simulink model "SF011A_EotLrng"  (R2013b)
settings: Solver=FixedStepDiscrete  SolverMode=SingleTasking  StartTime=0.0  StopTime=1  FixedStep=0.002  RelTol=1e-3
values from neighbouring files (symbols this model uses):
  ARCHGLBPRM_FLOATZEROTHD_ULS_F32 = DataDict.Constant    [SF011A_EotLrng_DataDict.m]
  CNVTOMILLISEC_MILLISECPERCNT_F32 = DataDict.Constant    [SF011A_EotLrng_DataDict.m]
  CORRLNFLT_CNT_U08 = DataDict.Constant    [SF011A_EotLrng_DataDict.m]
  DEBSTEP_CNT_U16 = DataDict.Constant    [SF011A_EotLrng_DataDict.m]
  EOTLIMDETD_CNT_LOGL = DataDict.Constant    [SF011A_EotLrng_DataDict.m]
  EOTLIMNOTDETD_CNT_LOGL = DataDict.Constant    [SF011A_EotLrng_DataDict.m]
  EotLrngAuthyStrtLrn = DataDict.Calibration    [SF011A_EotLrng_DataDict.m]
  EotLrngEotLrnTmr = DataDict.Calibration    [SF011A_EotLrng_DataDict.m]
  EotLrngHwAgOverTrvlCnt = DataDict.Calibration    [SF011A_EotLrng_DataDict.m]
  EotLrngHwAgOverTrvlEntr = DataDict.Calibration    [SF011A_EotLrng_DataDict.m]
  EotLrngHwAgOverTrvlExit = DataDict.Calibration    [SF011A_EotLrng_DataDict.m]
  EotLrngHwTqEotLrn = DataDict.Calibration    [SF011A_EotLrng_DataDict.m]
  EotLrngMotVelEotLrn = DataDict.Calibration    [SF011A_EotLrng_DataDict.m]
  EotLrngRackTrvlMax = DataDict.Calibration    [SF011A_EotLrng_DataDict.m]
  EotLrngRackTrvlMin = DataDict.Calibration    [SF011A_EotLrng_DataDict.m]
  EotLrngRstAuthyMin = DataDict.Calibration    [SF011A_EotLrng_DataDict.m]
  EotProtnRackTrvlLimrEna = DataDict.ImprtdCal    [SF011A_EotLrng_DataDict.m]
  HwAgOverTrvl = DataDict.NTC    [SF011A_EotLrng_DataDict.m]
  HWAGOVERTRVLMAXCNT_CNT_U08 = DataDict.Constant    [SF011A_EotLrng_DataDict.m]
  NODEBSTEP_CNT_U16 = DataDict.Constant    [SF011A_EotLrng_DataDict.m]
  OUTOFRNGFLT_CNT_U08 = DataDict.Constant    [SF011A_EotLrng_DataDict.m]
  RackEotStorgFlt = DataDict.NTC    [SF011A_EotLrng_DataDict.m]
  SIGAVLFLT_CNT_U08 = DataDict.Constant    [SF011A_EotLrng_DataDict.m]
undefined symbols (not defined in the file or in its folder): NtcSts1, NvmGetErrSts1, SigQlfr1
libraries: simulink x19, NxtrNvM x12, NxtrAbslt x5, NxtrLim x4, NxtrMax x3, NxtrMin x3
(part 2 of 7)

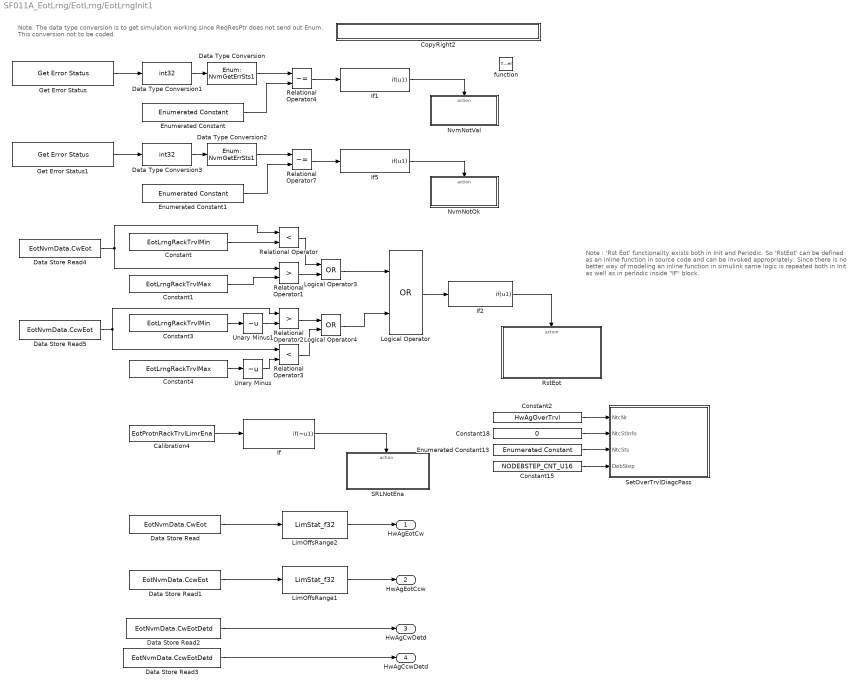
== system SF011A_EotLrng/EotLrng/EotLrngInit1 ==
  note: Note: The data type conversion is to get simulation working since ReqResPtr does not send out Enum. This
      | conversion not to be coded.
  note: Note : 'Rst Eot' functionality exists both in Init and Periodic.
      | So 'RstEot' can be defined as an inline function in source code and can be invoked
      | appropriately. Since there is no better way of modeling an inline function in simulink
      | same logic is repeated both in Init as well as in periodic inside "IF" block.
  function : TriggerPort  TriggerType=function-call
  Calibration4 : Constant  RequirementInfo="{'linktype_rmi_doors' '0000ba59 (/E-STEER Core/SubSystem Specifications/Application Functions/SF011A Learned EOT Limits)' '#SF011A_125' 'true' 'REQ:  SF011A_125' '' } %GIDa_8cd91484_508f_4a19_9e50_6e4bd6d6bfd9"  Value=EotProtnRackTrvlLimrEna
  Constant : Constant  RequirementInfo="{'linktype_rmi_doors' '0000ba59 (/E-STEER Core/SubSystem Specifications/Application Functions/SF011A Learned EOT Limits)' '#SF011A_70' 'true' 'REQ:  SF011A_70' '' ; 'linktype_rmi_doors' '0000ba59 (/E-STEER Core/SubSystem Specifications/Application Functions/SF011A Learned EOT Limits)' '#SF011A_48' 'true' 'REQ:  SF011A_48' '' } %GIDa_a6aa3c9d_e3af_4644_902f_5becbbdfb912"  Value=EotLrngRackTrvlMin
  Constant1 : Constant  RequirementInfo="{'linktype_rmi_doors' '0000ba59 (/E-STEER Core/SubSystem Specifications/Application Functions/SF011A Learned EOT Limits)' '#SF011A_70' 'true' 'REQ:  SF011A_70' '' ; 'linktype_rmi_doors' '0000ba59 (/E-STEER Core/SubSystem Specifications/Application Functions/SF011A Learned EOT Limits)' '#SF011A_49' 'true' 'REQ:  SF011A_49' '' } %GIDa_a0828fd1_c5cb_4d17_a3e1_4c408a8731ec"  Value=EotLrngRackTrvlMax
  Constant15 : Constant  RequirementInfo={} %GIDa_e57038bb_d9c8_49ea_a4b9_f6e761d5e128  Value=NODEBSTEP_CNT_U16
  Constant18 : Constant  RequirementInfo={} %GIDa_4611f9eb_ed4b_4f11_915a_23b80d8496d3  Value=0
  Constant2 : Constant  RequirementInfo={} %GIDa_c7caa921_f92d_4602_b505_ea668ad6087d  Value=HwAgOverTrvl
  Constant3 : Constant  RequirementInfo="{'linktype_rmi_doors' '0000ba59 (/E-STEER Core/SubSystem Specifications/Application Functions/SF011A Learned EOT Limits)' '#SF011A_71' 'true' 'REQ:  SF011A_71' '' ; 'linktype_rmi_doors' '0000ba59 (/E-STEER Core/SubSystem Specifications/Application Functions/SF011A Learned EOT Limits)' '#SF011A_48' 'true' 'REQ:  SF011A_48' '' } %GIDa_5f1678bd_b67c_4df4_9938_38fbe269600f"  Value=EotLrngRackTrvlMin
  Constant4 : Constant  RequirementInfo="{'linktype_rmi_doors' '0000ba59 (/E-STEER Core/SubSystem Specifications/Application Functions/SF011A Learned EOT Limits)' '#SF011A_71' 'true' 'REQ:  SF011A_71' '' ; 'linktype_rmi_doors' '0000ba59 (/E-STEER Core/SubSystem Specifications/Application Functions/SF011A Learned EOT Limits)' '#SF011A_49' 'true' 'REQ:  SF011A_49' '' } %GIDa_30774794_edea_413e_bdbc_5a0164b2a6d6"  Value=EotLrngRackTrvlMax
  CopyRight2 : Subsystem  Description=|  mask(Copyright Information){none=on}
      | Copyright info block.                                               
      |                                                                     
      | Place copyright information at the top of every subsystem in design.
      mask prompts: none "No parameters"
      mask help: Place copyright information at the top of every subsystem in design.
      mask Display:
      | NxtrConf = 'Nexteer Confidential';
      | 
      | sys = bdroot; %handle for the current model ("system")
      | first = get_param(sys,'Created');
      | if(isempty(first))
      |     first = datestr(now,'yyyy');
      | else
      |     first = first(end-3:end);  %year is last four digits
      | end
      | 
      | last = get_param(sys,'LastModifiedDate');
      | if isempty(last)
      |     last = datestr(now,'yyyy');
      | else
      |     last = last(end-3:end);
      | end
      | 
      | if strcmp(first,last)
      |     fprintf('%s -- Copyright %s Nexteer',NxtrConf,first)
      | else
      |     fprintf('%s -- %s%s- %s Nexteer',NxtrConf,char(169),first,last)
      | end
  Data Store Read : DataStoreRead  RequirementInfo="{'linktype_rmi_doors' '0000ba59 (/E-STEER Core/SubSystem Specifications/Application Functions/SF011A Learned EOT Limits)' '#SF011A_60' 'true' 'REQ:  SF011A_60' '' ; 'linktype_rmi_doors' '0000ba59 (/E-STEER Core/SubSystem Specifications/Application Functions/SF011A Learned EOT Limits)' '#SF011A_59' 'true' 'REQ:  SF011A_59' '' ; 'linktype_rmi_doors' '0000ba59 (/E-STEER Core/SubSystem Specifications/Application Functions/SF011A Learned EOT Limits)' '#SF011A_72' 'true' 'REQ:  SF011A_72' '' } %GIDa_1cce3593_98c7_4927_96ef_8fd09f8c13ce"  DataStoreName=EotNvmData  DataStoreElements=EotNvmData.CwEot
  Data Store Read1 : DataStoreRead  RequirementInfo="{'linktype_rmi_doors' '0000ba59 (/E-STEER Core/SubSystem Specifications/Application Functions/SF011A Learned EOT Limits)' '#SF011A_61' 'true' 'REQ:  SF011A_61' '' ; 'linktype_rmi_doors' '0000ba59 (/E-STEER Core/SubSystem Specifications/Application Functions/SF011A Learned EOT Limits)' '#SF011A_59' 'true' 'REQ:  SF011A_59' '' ; 'linktype_rmi_doors' '0000ba59 (/E-STEER Core/SubSystem Specifications/Application Functions/SF011A Learned EOT Limits)' '#SF011A_73' 'true' 'REQ:  SF011A_73' '' } %GIDa_59ef2486_936c_413c_9940_c67c54ecfdbd"  DataStoreName=EotNvmData  DataStoreElements=EotNvmData.CcwEot
  Data Store Read2 : DataStoreRead  RequirementInfo="{'linktype_rmi_doors' '0000ba59 (/E-STEER Core/SubSystem Specifications/Application Functions/SF011A Learned EOT Limits)' '#SF011A_62' 'true' 'REQ:  SF011A_62' '' ; 'linktype_rmi_doors' '0000ba59 (/E-STEER Core/SubSystem Specifications/Application Functions/SF011A Learned EOT Limits)' '#SF011A_59' 'true' 'REQ:  SF011A_59' '' ; 'linktype_rmi_doors' '0000ba59 (/E-STEER Core/SubSystem Specifications/Application Functions/SF011A Learned EOT Limits)' '#SF011A_74' 'true' 'REQ:  SF011A_74' '' } %GIDa_37d3043a_15c7_4be1_94c6_67c59661e3c0"  DataStoreName=EotNvmData  DataStoreElements=EotNvmData.CwEotDetd
  Data Store Read3 : DataStoreRead  RequirementInfo="{'linktype_rmi_doors' '0000ba59 (/E-STEER Core/SubSystem Specifications/Application Functions/SF011A Learned EOT Limits)' '#SF011A_63' 'true' 'REQ:  SF011A_63' '' ; 'linktype_rmi_doors' '0000ba59 (/E-STEER Core/SubSystem Specifications/Application Functions/SF011A Learned EOT Limits)' '#SF011A_59' 'true' 'REQ:  SF011A_59' '' ; 'linktype_rmi_doors' '0000ba59 (/E-STEER Core/SubSystem Specifications/Application Functions/SF011A Learned EOT Limits)' '#SF011A_75' 'true' 'REQ:  SF011A_75' '' } %GIDa_cb0e143f_3fff_4146_ad36_117712b20001"  DataStoreName=EotNvmData  DataStoreElements=EotNvmData.CcwEotDetd
  Data Store Read4 : DataStoreRead  RequirementInfo="{'linktype_rmi_doors' '0000ba59 (/E-STEER Core/SubSystem Specifications/Application Functions/SF011A Learned EOT Limits)' '#SF011A_70' 'true' 'REQ:  SF011A_70' '' } %GIDa_1f2eef30_41ac_4ca5_aa34_dae99e9f45ec"  DataStoreName=EotNvmData  DataStoreElements=EotNvmData.CwEot
  Data Store Read5 : DataStoreRead  RequirementInfo="{'linktype_rmi_doors' '0000ba59 (/E-STEER Core/SubSystem Specifications/Application Functions/SF011A Learned EOT Limits)' '#SF011A_71' 'true' 'REQ:  SF011A_71' '' } %GIDa_ec91acdb_3367_426b_b3a6_fca3d2bebdb1"  DataStoreName=EotNvmData  DataStoreElements=EotNvmData.CcwEot
  Data Type Conversion : DataTypeConversion  RequirementInfo="{'linktype_rmi_doors' '0000ba59 (/E-STEER Core/SubSystem Specifications/Application Functions/SF011A Learned EOT Limits)' '#SF011A_124' 'true' 'REQ:  SF011A_124' '' } %GIDa_40e4bb70_1115_4c40_912d_1afd6378f698"  OutDataTypeStr=Enum: NvmGetErrSts1
  Data Type Conversion1 : DataTypeConversion  RequirementInfo="{'linktype_rmi_doors' '0000ba59 (/E-STEER Core/SubSystem Specifications/Application Functions/SF011A Learned EOT Limits)' '#SF011A_124' 'true' 'REQ:  SF011A_124' '' } %GIDa_af9c1c5f_4576_4c81_a62f_597d688de759"  OutDataTypeStr=int32
  Data Type Conversion2 : DataTypeConversion  RequirementInfo="{'linktype_rmi_doors' '0000ba59 (/E-STEER Core/SubSystem Specifications/Application Functions/SF011A Learned EOT Limits)' '#SF011A_124' 'true' 'REQ:  SF011A_124' '' } %GIDa_9c8c0f48_10fc_41fa_ac24_1a39867ed0ea"  OutDataTypeStr=Enum: NvmGetErrSts1
  Data Type Conversion3 : DataTypeConversion  RequirementInfo="{'linktype_rmi_doors' '0000ba59 (/E-STEER Core/SubSystem Specifications/Application Functions/SF011A Learned EOT Limits)' '#SF011A_124' 'true' 'REQ:  SF011A_124' '' } %GIDa_ea8dac4b_68c0_40a2_8dd8_c1010ce976e9"  OutDataTypeStr=int32
  Enumerated Constant13 : simulink/Sources/Enumerated Constant  RequirementInfo={} %GIDa_38909906_b1fb_4b03_8f37_3dee4a706b69  OutDataTypeStr=Enum: NtcSts1  Value=NtcSts1.NTCSTS_PASSD  SampleTime=inf
  Enumerated Constant : simulink/Sources/Enumerated Constant  RequirementInfo="{'linktype_rmi_doors' '0000ba59 (/E-STEER Core/SubSystem Specifications/Application Functions/SF011A Learned EOT Limits)' '#SF011A_124' 'true' 'REQ:  SF011A_124' '' } %GIDa_af7030e8_a7a1_47be_8aa5_0a8feabfae11"  OutDataTypeStr=Enum: NvmGetErrSts1  Value=NvmGetErrSts1.REQUEST_OK  SampleTime=inf
  Enumerated Constant1 : simulink/Sources/Enumerated Constant  RequirementInfo="{'linktype_rmi_doors' '0000ba59 (/E-STEER Core/SubSystem Specifications/Application Functions/SF011A Learned EOT Limits)' '#SF011A_124' 'true' 'REQ:  SF011A_124' '' } %GIDa_38a139b3_f8e9_4563_8a22_5346e1b58213"  OutDataTypeStr=Enum: NvmGetErrSts1  Value=NvmGetErrSts1.REQUEST_OK  SampleTime=inf
  Get Error Status : NxtrNvM/Get Error Status  RequirementInfo="{'linktype_rmi_doors' '0000ba59 (/E-STEER Core/SubSystem Specifications/Application Functions/SF011A Learned EOT Limits)' '#SF011A_124' 'true' 'REQ:  SF011A_124' '' } %GIDa_295c35b2_dd27_46e5_9350_5c6db25722f0"  FuncName=Get Error Status  NvMBlockName=EotNvmData  VoidFuncRtn=on  ReqResPtr_DSN=NvMReqResPtr  Return_DSN=NvMGES_ReqResPtr
      settings: AttributesFormatString=%<FuncName>
  Get Error Status1 : NxtrNvM/Get Error Status  RequirementInfo="{'linktype_rmi_doors' '0000ba59 (/E-STEER Core/SubSystem Specifications/Application Functions/SF011A Learned EOT Limits)' '#SF011A_124' 'true' 'REQ:  SF011A_124' '' } %GIDa_5993ad55_5530_455e_9e47_61c827e0bbdf"  FuncName=Get Error Status  NvMBlockName=MaxHwAgCwAndCcw  VoidFuncRtn=on  ReqResPtr_DSN=NvMReqResPtr1  Return_DSN=NvMGES_ReqResPtr1
      settings: AttributesFormatString=%<FuncName>
  If : If  RequirementInfo="{'linktype_rmi_doors' '0000ba59 (/E-STEER Core/SubSystem Specifications/Application Functions/SF011A Learned EOT Limits)' '#SF011A_125' 'true' 'REQ:  SF011A_125' '' } %GIDa_3d6ad9bb_5e78_4a41_a61b_bd13d670cab6"  Priority=2  IfExpression=~u1  ShowElse=off
  If1 : If  RequirementInfo="{'linktype_rmi_doors' '0000ba59 (/E-STEER Core/SubSystem Specifications/Application Functions/SF011A Learned EOT Limits)' '#SF011A_124' 'true' 'REQ:  SF011A_124' '' } %GIDa_91d6c890_e003_4682_8730_094d0138a595"  Priority=0  IfExpression=u1  ShowElse=off
  If2 : If  RequirementInfo="{'linktype_rmi_doors' '0000ba59 (/E-STEER Core/SubSystem Specifications/Application Functions/SF011A Learned EOT Limits)' '#SF011A_70' 'true' 'REQ:  SF011A_70' '' ; 'linktype_rmi_doors' '0000ba59 (/E-STEER Core/SubSystem Specifications/Application Functions/SF011A Learned EOT Limits)' '#SF011A_71' 'true' 'REQ:  SF011A_71' '' } %GIDa_a534ff47_bac3_4be0_88f9_462c603ec428"  Priority=1  IfExpression=u1  ShowElse=off
  If5 : If  RequirementInfo="{'linktype_rmi_doors' '0000ba59 (/E-STEER Core/SubSystem Specifications/Application Functions/SF011A Learned EOT Limits)' '#SF011A_124' 'true' 'REQ:  SF011A_124' '' } %GIDa_8f477629_7324_4566_aadd_9e30a62de6d3"  Priority=0  IfExpression=u1  ShowElse=off
  LimOffsRange1 : NxtrLim/LimStat_f32  RequirementInfo="{'linktype_rmi_doors' '0000ba59 (/E-STEER Core/SubSystem Specifications/Application Functions/SF011A Learned EOT Limits)' '#SF011A_39' 'true' 'REQ:  SF011A_39' '' } %GIDa_51d5d642_7edf_4836_a1f4_3c017c910443"  LoLim=HWAGEOTCCWLOWLIM_HWDEG_F32  HiLim=HWAGEOTCCWHILIM_HWDEG_F32
      settings: AttributesFormatString=|
      | Low Limit: %<LoLim>
      | High Limit:%<HiLim>
  LimOffsRange2 : NxtrLim/LimStat_f32  RequirementInfo="{'linktype_rmi_doors' '0000ba59 (/E-STEER Core/SubSystem Specifications/Application Functions/SF011A Learned EOT Limits)' '#SF011A_11' 'true' 'REQ:  SF011A_11' '' } %GIDa_4df0df7c_5c40_4811_b091_ccf12396757f"  LoLim=HWAGEOTCWLOWLIM_HWDEG_F32  HiLim=HWAGEOTCWHILIM_HWDEG_F32
      settings: AttributesFormatString=|
      | Low Limit: %<LoLim>
      | High Limit:%<HiLim>
  Logical Operator : Logic  RequirementInfo="{'linktype_rmi_doors' '0000ba59 (/E-STEER Core/SubSystem Specifications/Application Functions/SF011A Learned EOT Limits)' '#SF011A_70' 'true' 'REQ:  SF011A_70' '' ; 'linktype_rmi_doors' '0000ba59 (/E-STEER Core/SubSystem Specifications/Application Functions/SF011A Learned EOT Limits)' '#SF011A_71' 'true' 'REQ:  SF011A_71' '' } %GIDa_ebb98ba6_f107_46ce_9d07_fa346759ea33"  Operator=OR  AllPortsSameDT=off  OutDataTypeStr=boolean
  Logical Operator3 : Logic  RequirementInfo="{'linktype_rmi_doors' '0000ba59 (/E-STEER Core/SubSystem Specifications/Application Functions/SF011A Learned EOT Limits)' '#SF011A_70' 'true' 'REQ:  SF011A_70' '' } %GIDa_aaf30ec3_ce61_43e6_b06a_936d4bd8ccf6"  Operator=OR  AllPortsSameDT=off  OutDataTypeStr=boolean
  Logical Operator4 : Logic  RequirementInfo="{'linktype_rmi_doors' '0000ba59 (/E-STEER Core/SubSystem Specifications/Application Functions/SF011A Learned EOT Limits)' '#SF011A_71' 'true' 'REQ:  SF011A_71' '' } %GIDa_33792c4b_275f_4e69_ac68_2ae50f8c8a65"  Operator=OR  AllPortsSameDT=off  OutDataTypeStr=boolean
  NvmNotOk : Subsystem  RequirementInfo="{'linktype_rmi_doors' '0000ba59 (/E-STEER Core/SubSystem Specifications/Application Functions/SF011A Learned EOT Limits)' '#SF011A_124' 'true' 'REQ:  SF011A_124' '' } %GIDa_4462a29b_32ac_4e56_9b35_32a96dafcb01"  TreatAsAtomicUnit=on
  NvmNotVal : Subsystem  RequirementInfo="{'linktype_rmi_doors' '0000ba59 (/E-STEER Core/SubSystem Specifications/Application Functions/SF011A Learned EOT Limits)' '#SF011A_124' 'true' 'REQ:  SF011A_124' '' } %GIDa_0aa83e4c_487d_4e38_aff6_7f3e0cc4b065"  TreatAsAtomicUnit=on
  Relational Operator : RelationalOperator  RequirementInfo="{'linktype_rmi_doors' '0000ba59 (/E-STEER Core/SubSystem Specifications/Application Functions/SF011A Learned EOT Limits)' '#SF011A_70' 'true' 'REQ:  SF011A_70' '' } %GIDa_5740cdc3_fa46_4f68_ba56_8a0600b2e95d"  Operator=<  OutDataTypeStr=boolean
  Relational Operator1 : RelationalOperator  RequirementInfo="{'linktype_rmi_doors' '0000ba59 (/E-STEER Core/SubSystem Specifications/Application Functions/SF011A Learned EOT Limits)' '#SF011A_70' 'true' 'REQ:  SF011A_70' '' } %GIDa_6b96990d_fede_45f3_8f31_228d4b94cd2a"  Operator=>  OutDataTypeStr=boolean
  Relational Operator2 : RelationalOperator  RequirementInfo="{'linktype_rmi_doors' '0000ba59 (/E-STEER Core/SubSystem Specifications/Application Functions/SF011A Learned EOT Limits)' '#SF011A_71' 'true' 'REQ:  SF011A_71' '' } %GIDa_42bd1801_e5df_4c76_b346_5582a84dc674"  Operator=>  OutDataTypeStr=boolean
  Relational Operator3 : RelationalOperator  RequirementInfo="{'linktype_rmi_doors' '0000ba59 (/E-STEER Core/SubSystem Specifications/Application Functions/SF011A Learned EOT Limits)' '#SF011A_71' 'true' 'REQ:  SF011A_71' '' } %GIDa_a5e949b1_27bf_4f78_b47a_8cc68d8ee70e"  Operator=<  OutDataTypeStr=boolean
  Relational Operator4 : RelationalOperator  RequirementInfo="{'linktype_rmi_doors' '0000ba59 (/E-STEER Core/SubSystem Specifications/Application Functions/SF011A Learned EOT Limits)' '#SF011A_124' 'true' 'REQ:  SF011A_124' '' } %GIDa_19950154_b903_4425_aebc_606c335bc66e"  Operator=~=  OutDataTypeStr=boolean
  Relational Operator7 : RelationalOperator  RequirementInfo="{'linktype_rmi_doors' '0000ba59 (/E-STEER Core/SubSystem Specifications/Application Functions/SF011A Learned EOT Limits)' '#SF011A_124' 'true' 'REQ:  SF011A_124' '' } %GIDa_6f49dc21_33c5_4733_8830_c8a8f380ec87"  Operator=~=  OutDataTypeStr=boolean
  RstEot : Subsystem  RequirementInfo="{'linktype_rmi_doors' '0000ba59 (/E-STEER Core/SubSystem Specifications/Application Functions/SF011A Learned EOT Limits)' '#SF011A_70' 'true' 'REQ:  SF011A_70' '' ; 'linktype_rmi_doors' '0000ba59 (/E-STEER Core/SubSystem Specifications/Application Functions/SF011A Learned EOT Limits)' '#SF011A_71' 'true' 'REQ:  SF011A_71' '' ; 'linktype_rmi_doors' '0000ba59 (/E-STEER Core/SubSystem Specifications/Application Functions/SF011A Learned EOT Limits)' '#SF011A_64' 'true' 'REQ:  SF011A_64' '' } %GIDa_e945f950_1b9a_4a4b_872f_96aafbb976bf"  TreatAsAtomicUnit=on
  SRLNotEna : Subsystem  RequirementInfo="{'linktype_rmi_doors' '0000ba59 (/E-STEER Core/SubSystem Specifications/Application Functions/SF011A Learned EOT Limits)' '#SF011A_125' 'true' 'REQ:  SF011A_125' '' } %GIDa_fcf323af_a30f_442e_9919_a2f8c84ea324"  TreatAsAtomicUnit=on
  SetOverTrvlDiagcPass : Subsystem  RequirementInfo="{'linktype_rmi_doors' '0000ba59 (/E-STEER Core/SubSystem Specifications/Application Functions/SF011A Learned EOT Limits)' '#SF011A_207' 'true' 'REQ:  SF011A_207' '' } %GIDa_e6b84ba3_d050_4a47_96a0_b05ce6a68eb1"  mask(SetNTC){}
      mask help: SetNTC library block
  Unary Minus : UnaryMinus  RequirementInfo="{'linktype_rmi_doors' '0000ba59 (/E-STEER Core/SubSystem Specifications/Application Functions/SF011A Learned EOT Limits)' '#SF011A_71' 'true' 'REQ:  SF011A_71' '' } %GIDa_83e2cf92_ba7d_4967_a036_f97e746d9f9d"
  Unary Minus1 : UnaryMinus  RequirementInfo="{'linktype_rmi_doors' '0000ba59 (/E-STEER Core/SubSystem Specifications/Application Functions/SF011A Learned EOT Limits)' '#SF011A_71' 'true' 'REQ:  SF011A_71' '' } %GIDa_4ca99ef1_4085_4f91_be59_96051a391331"
  HwAgEotCw : Outport  RequirementInfo="{'linktype_rmi_doors' '0000ba59 (/E-STEER Core/SubSystem Specifications/Application Functions/SF011A Learned EOT Limits)' '#SF011A_59' 'true' 'REQ:  SF011A_59' '' ; 'linktype_rmi_doors' '0000ba59 (/E-STEER Core/SubSystem Specifications/Application Functions/SF011A Learned EOT Limits)' '#SF011A_60' 'true' 'REQ:  SF011A_60' '' ; 'linktype_rmi_doors' '0000ba59 (/E-STEER Core/SubSystem Specifications/Application Functions/SF011A Learned EOT Limits)' '#SF011A_72' 'true' 'REQ:  SF011A_72' '' } %GIDa_4d8ef3fe_5383_4a70_a8ac_cac3ef6a99ba"
  HwAgEotCcw : Outport  RequirementInfo="{'linktype_rmi_doors' '0000ba59 (/E-STEER Core/SubSystem Specifications/Application Functions/SF011A Learned EOT Limits)' '#SF011A_59' 'true' 'REQ:  SF011A_59' '' ; 'linktype_rmi_doors' '0000ba59 (/E-STEER Core/SubSystem Specifications/Application Functions/SF011A Learned EOT Limits)' '#SF011A_61' 'true' 'REQ:  SF011A_61' '' ; 'linktype_rmi_doors' '0000ba59 (/E-STEER Core/SubSystem Specifications/Application Functions/SF011A Learned EOT Limits)' '#SF011A_73' 'true' 'REQ:  SF011A_73' '' } %GIDa_597d9c11_d72e_4b97_8dbc_75152cd21626"  Port=2
  HwAgCwDetd : Outport  RequirementInfo="{'linktype_rmi_doors' '0000ba59 (/E-STEER Core/SubSystem Specifications/Application Functions/SF011A Learned EOT Limits)' '#SF011A_59' 'true' 'REQ:  SF011A_59' '' ; 'linktype_rmi_doors' '0000ba59 (/E-STEER Core/SubSystem Specifications/Application Functions/SF011A Learned EOT Limits)' '#SF011A_62' 'true' 'REQ:  SF011A_62' '' ; 'linktype_rmi_doors' '0000ba59 (/E-STEER Core/SubSystem Specifications/Application Functions/SF011A Learned EOT Limits)' '#SF011A_74' 'true' 'REQ:  SF011A_74' '' } %GIDa_82c8644a_2e69_4c9e_99fb_f95f059f9627"  Port=3
  HwAgCcwDetd : Outport  RequirementInfo="{'linktype_rmi_doors' '0000ba59 (/E-STEER Core/SubSystem Specifications/Application Functions/SF011A Learned EOT Limits)' '#SF011A_59' 'true' 'REQ:  SF011A_59' '' ; 'linktype_rmi_doors' '0000ba59 (/E-STEER Core/SubSystem Specifications/Application Functions/SF011A Learned EOT Limits)' '#SF011A_63' 'true' 'REQ:  SF011A_63' '' ; 'linktype_rmi_doors' '0000ba59 (/E-STEER Core/SubSystem Specifications/Application Functions/SF011A Learned EOT Limits)' '#SF011A_75' 'true' 'REQ:  SF011A_75' '' } %GIDa_50a9f717_3ffd_4e5e_8c83_459633dce401"  Port=4
  wires:
  If1/1 -> NvmNotVal/Action
  Relational Operator4/1 -> If1/1
  Data Store Read4/1 -> Relational Operator1/1, Relational Operator/1
  Logical Operator/1 -> If2/1
  If2/1 -> RstEot/Action
  Constant/1 -> Relational Operator/2
  Constant1/1 -> Relational Operator1/2
  Relational Operator/1 -> Logical Operator3/1
  Relational Operator1/1 -> Logical Operator3/2
  Logical Operator3/1 -> Logical Operator/1
  Data Store Read5/1 -> Relational Operator3/1, Relational Operator2/1
  Constant3/1 -> Unary Minus1/1
  Constant4/1 -> Unary Minus/1
  Unary Minus/1 -> Relational Operator3/2
  Unary Minus1/1 -> Relational Operator2/2
  Relational Operator2/1 -> Logical Operator4/1
  Relational Operator3/1 -> Logical Operator4/2
  Logical Operator4/1 -> Logical Operator/2
  Calibration4/1 -> If/1
  If/1 -> SRLNotEna/Action
  Enumerated Constant/1 -> Relational Operator4/2
  Data Type Conversion/1 -> Relational Operator4/1
  Get Error Status/1 -> Data Type Conversion1/1
  Data Type Conversion1/1 -> Data Type Conversion/1
  Data Store Read/1 -> LimOffsRange2/1
  Data Store Read1/1 -> LimOffsRange1/1
  Data Store Read2/1 -> HwAgCwDetd/1
  Data Store Read3/1 -> HwAgCcwDetd/1
  LimOffsRange2/1 -> HwAgEotCw/1
  LimOffsRange1/1 -> HwAgEotCcw/1
  If5/1 -> NvmNotOk/Action
  Relational Operator7/1 -> If5/1
  Enumerated Constant1/1 -> Relational Operator7/2
  Data Type Conversion2/1 -> Relational Operator7/1
  Get Error Status1/1 -> Data Type Conversion3/1
  Data Type Conversion3/1 -> Data Type Conversion2/1
  Constant15/1 -> SetOverTrvlDiagcPass/4(DebStep)
  Enumerated Constant13/1 -> SetOverTrvlDiagcPass/3(NtcSts)
  Constant18/1 -> SetOverTrvlDiagcPass/2(NtcStInfo)
  Constant2/1 -> SetOverTrvlDiagcPass/1(NtcNr)

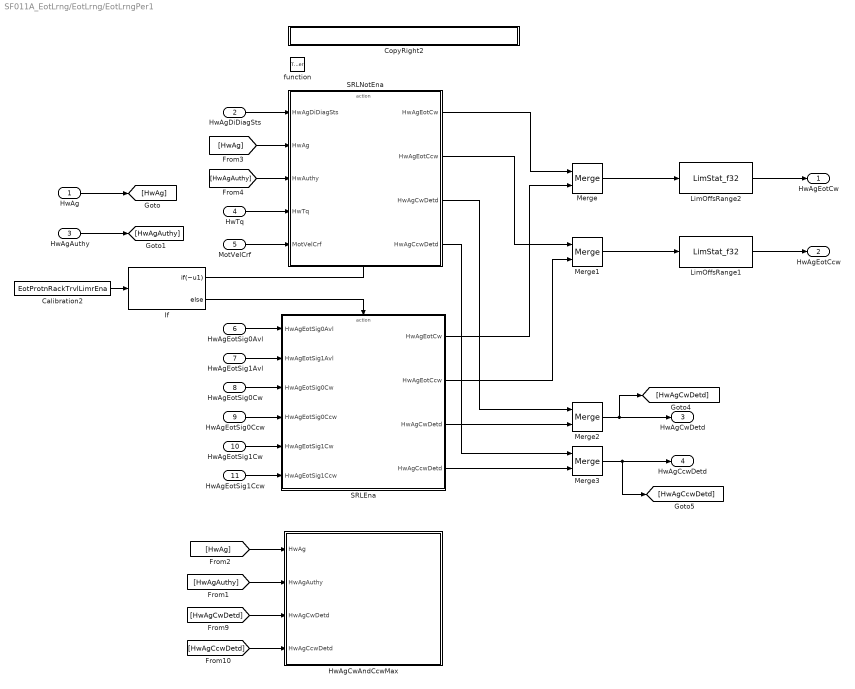
== system SF011A_EotLrng/EotLrng/EotLrngPer1 ==
  HwAg : Inport  RequirementInfo={} %GIDa_b4cee634_5ee9_4149_9ddf_f8cff9cb8062
  HwAgDiDiagSts : Inport  Port=2
  HwAgAuthy : Inport  Port=3
  HwTq : Inport  Port=4
  MotVelCrf : Inport  Port=5
  HwAgEotSig0Avl : Inport  Port=6
  HwAgEotSig1Avl : Inport  Port=7
  HwAgEotSig0Cw : Inport  Port=8
  HwAgEotSig0Ccw : Inport  Port=9
  HwAgEotSig1Cw : Inport  Port=10
  HwAgEotSig1Ccw : Inport  Port=11
  function : TriggerPort  TriggerType=function-call
  Calibration2 : Constant  RequirementInfo="{'linktype_rmi_doors' '0000ba59 (/E-STEER Core/SubSystem Specifications/Application Functions/SF011A Learned EOT Limits)' '#SF011A_119' 'true' 'REQ:  SF011A_119' '' } %GIDa_0b0ed5cd_7684_4e3d_b855_9f34f3ebafd9"  Value=EotProtnRackTrvlLimrEna
  CopyRight2 : Subsystem  Description=|  mask(Copyright Information){none=on}
      | Copyright info block.                                               
      |                                                                     
      | Place copyright information at the top of every subsystem in design.
      mask prompts: none "No parameters"
      mask help: Place copyright information at the top of every subsystem in design.
      mask Display:
      | NxtrConf = 'Nexteer Confidential';
      | 
      | sys = bdroot; %handle for the current model ("system")
      | first = get_param(sys,'Created');
      | if(isempty(first))
      |     first = datestr(now,'yyyy');
      | else
      |     first = first(end-3:end);  %year is last four digits
      | end
      | 
      | last = get_param(sys,'LastModifiedDate');
      | if isempty(last)
      |     last = datestr(now,'yyyy');
      | else
      |     last = last(end-3:end);
      | end
      | 
      | if strcmp(first,last)
      |     fprintf('%s -- Copyright %s Nexteer',NxtrConf,first)
      | else
      |     fprintf('%s -- %s%s- %s Nexteer',NxtrConf,char(169),first,last)
      | end
  HwAgCwAndCcwMax : Subsystem
  If : If  RequirementInfo="{'linktype_rmi_doors' '0000ba59 (/E-STEER Core/SubSystem Specifications/Application Functions/SF011A Learned EOT Limits)' '#SF011A_128' 'true' 'REQ:  SF011A_128' '' ; 'linktype_rmi_doors' '0000ba59 (/E-STEER Core/SubSystem Specifications/Application Functions/SF011A Learned EOT Limits)' '#SF011A_143' 'true' 'REQ:  SF011A_143' '' ; 'linktype_rmi_doors' '0000ba59 (/E-STEER Core/SubSystem Specifications/Application Functions/SF011A Learned EOT Limits)' '#SF011A_119' 'true' 'REQ:  SF011A_119' '' } %GIDa_a7d7eb2f_b2f2_41f0_8f1a_6ef2ae590523"  Priority=0  IfExpression=~u1
  LimOffsRange1 : NxtrLim/LimStat_f32  LoLim=HWAGEOTCCWLOWLIM_HWDEG_F32  HiLim=HWAGEOTCCWHILIM_HWDEG_F32
      settings: AttributesFormatString=|
      | Low Limit: %<LoLim>
      | High Limit:%<HiLim>
  LimOffsRange2 : NxtrLim/LimStat_f32  LoLim=HWAGEOTCWLOWLIM_HWDEG_F32  HiLim=HWAGEOTCWHILIM_HWDEG_F32
      settings: AttributesFormatString=|
      | Low Limit: %<LoLim>
      | High Limit:%<HiLim>
  Merge{,1..3} (4 alike) : Merge
  SRLEna : Subsystem  RequirementInfo="{'linktype_rmi_doors' '0000ba59 (/E-STEER Core/SubSystem Specifications/Application Functions/SF011A Learned EOT Limits)' '#SF011A_119' 'true' 'REQ:  SF011A_119' '' } %GIDa_a05b4dc7_a6bb_4090_abea_45afd92bdff1"  TreatAsAtomicUnit=on
  SRLNotEna : Subsystem  RequirementInfo="{'linktype_rmi_doors' '0000ba59 (/E-STEER Core/SubSystem Specifications/Application Functions/SF011A Learned EOT Limits)' '#SF011A_119' 'true' 'REQ:  SF011A_119' '' ; 'linktype_rmi_doors' '0000ba59 (/E-STEER Core/SubSystem Specifications/Application Functions/SF011A Learned EOT Limits)' '#SF011A_128' 'true' 'REQ:  SF011A_128' '' } %GIDa_dde62c0f_30bf_4bd5_a1f9_116a11420e64"  TreatAsAtomicUnit=on
  HwAgEotCw : Outport
  HwAgEotCcw : Outport  Port=2
  HwAgCwDetd : Outport  Port=3
  HwAgCcwDetd : Outport  Port=4
  wires:
  If/1 -> SRLNotEna/Action
  Calibration2/1 -> If/1
  HwTq/1 -> SRLNotEna/4(HwTq)
  MotVelCrf/1 -> SRLNotEna/5(MotVelCrf)
  HwAgDiDiagSts/1 -> SRLNotEna/1(HwAgDiDiagSts)
  [HwAg] -> SRLNotEna/2(HwAg)
  [HwAgAuthy] -> SRLNotEna/3(HwAuthy)
  HwAgEotSig0Avl/1 -> SRLEna/1(HwAgEotSig0Avl)
  HwAgEotSig1Avl/1 -> SRLEna/2(HwAgEotSig1Avl)
  HwAgEotSig0Cw/1 -> SRLEna/3(HwAgEotSig0Cw)
  HwAgEotSig0Ccw/1 -> SRLEna/4(HwAgEotSig0Ccw)
  HwAgEotSig1Cw/1 -> SRLEna/5(HwAgEotSig1Cw)
  HwAgEotSig1Ccw/1 -> SRLEna/6(HwAgEotSig1Ccw)
  If/2 -> SRLEna/Action
  LimOffsRange2/1 -> HwAgEotCw/1
  LimOffsRange1/1 -> HwAgEotCcw/1
  SRLNotEna/1(HwAgEotCw) -> Merge/1
  SRLEna/1(HwAgEotCw) -> Merge/2
  SRLNotEna/2(HwAgEotCcw) -> Merge1/1
  SRLEna/2(HwAgEotCcw) -> Merge1/2
  SRLNotEna/3(HwAgCwDetd) -> Merge2/1
  SRLEna/3(HwAgCwDetd) -> Merge2/2
  SRLNotEna/4(HwAgCcwDetd) -> Merge3/1
  SRLEna/4(HwAgCcwDetd) -> Merge3/2
  HwAg/1 -> [HwAg]
  [HwAg] -> HwAgCwAndCcwMax/1(HwAg)
  HwAgAuthy/1 -> [HwAgAuthy]
  [HwAgAuthy] -> HwAgCwAndCcwMax/2(HwAgAuthy)
  Merge/1 -> LimOffsRange2/1
  Merge1/1 -> LimOffsRange1/1
  Merge2/1 -> [HwAgCwDetd], HwAgCwDetd/1
  Merge3/1 -> [HwAgCcwDetd], HwAgCcwDetd/1
  [HwAgCwDetd] -> HwAgCwAndCcwMax/3(HwAgCwDetd)
  [HwAgCcwDetd] -> HwAgCwAndCcwMax/4(HwAgCcwDetd)

== system SF011A_EotLrng/EotLrng/GetHwAgOverTrvlCnt ==
  function : TriggerPort  TriggerType=function-call
  CopyRight2 : Subsystem  Description=|  mask(Copyright Information){none=on}
      | Copyright info block.                                               
      |                                                                     
      | Place copyright information at the top of every subsystem in design.
      mask prompts: none "No parameters"
      mask help: Place copyright information at the top of every subsystem in design.
      mask Display:
      | NxtrConf = 'Nexteer Confidential';
      | 
      | sys = bdroot; %handle for the current model ("system")
      | first = get_param(sys,'Created');
      | if(isempty(first))
      |     first = datestr(now,'yyyy');
      | else
      |     first = first(end-3:end);  %year is last four digits
      | end
      | 
      | last = get_param(sys,'LastModifiedDate');
      | if isempty(last)
      |     last = datestr(now,'yyyy');
      | else
      |     last = last(end-3:end);
      | end
      | 
      | if strcmp(first,last)
      |     fprintf('%s -- Copyright %s Nexteer',NxtrConf,first)
      | else
      |     fprintf('%s -- %s%s- %s Nexteer',NxtrConf,char(169),first,last)
      | end
  Data Store Read : DataStoreRead  RequirementInfo="{'linktype_rmi_doors' '0000ba59 (/E-STEER Core/SubSystem Specifications/Application Functions/SF011A Learned EOT Limits)' '#SF011A_204' 'true' 'REQ:  SF011A_204' '' } %GIDa_dc99b738_73f2_41fb_92e1_a837c28f0398"  DataStoreName=MaxHwAgCwAndCcw  DataStoreElements=MaxHwAgCwAndCcw.HwAgOverTrvlCnt
  HwAgOverTrvlCnt : Outport  RequirementInfo="{'linktype_rmi_doors' '0000ba59 (/E-STEER Core/SubSystem Specifications/Application Functions/SF011A Learned EOT Limits)' '#SF011A_204' 'true' 'REQ:  SF011A_204' '' } %GIDa_07d13d9a_9d37_4eb9_aacf_190065f13365"
  wires:
  Data Store Read/1 -> HwAgOverTrvlCnt/1

== system SF011A_EotLrng/EotLrng/RstHwAgOverTrvlCnt ==
  function : TriggerPort  TriggerType=function-call
  " " : Constant  RequirementInfo="{'linktype_rmi_doors' '0000ba59 (/E-STEER Core/SubSystem Specifications/Application Functions/SF011A Learned EOT Limits)' '#SF011A_196' 'true' 'REQ:  SF011A_196' '' } %GIDa_af3f2046_743f_44fa_a7a3_d1909afda68c"  Value=0  OutDataTypeStr=uint8
      settings: AttributesFormatString=%<OutDataTypeStr>
  CopyRight2 : Subsystem  Description=|  mask(Copyright Information){none=on}
      | Copyright info block.                                               
      |                                                                     
      | Place copyright information at the top of every subsystem in design.
      mask prompts: none "No parameters"
      mask help: Place copyright information at the top of every subsystem in design.
      mask Display:
      | NxtrConf = 'Nexteer Confidential';
      | 
      | sys = bdroot; %handle for the current model ("system")
      | first = get_param(sys,'Created');
      | if(isempty(first))
      |     first = datestr(now,'yyyy');
      | else
      |     first = first(end-3:end);  %year is last four digits
      | end
      | 
      | last = get_param(sys,'LastModifiedDate');
      | if isempty(last)
      |     last = datestr(now,'yyyy');
      | else
      |     last = last(end-3:end);
      | end
      | 
      | if strcmp(first,last)
      |     fprintf('%s -- Copyright %s Nexteer',NxtrConf,first)
      | else
      |     fprintf('%s -- %s%s- %s Nexteer',NxtrConf,char(169),first,last)
      | end
  Data Store Write : DataStoreWrite  RequirementInfo="{'linktype_rmi_doors' '0000ba59 (/E-STEER Core/SubSystem Specifications/Application Functions/SF011A Learned EOT Limits)' '#SF011A_196' 'true' 'REQ:  SF011A_196' '' } %GIDa_41c4bb7c_ca45_4999_a871_c5bf0a758a42"  DataStoreName=MaxHwAgCwAndCcw  DataStoreElements=MaxHwAgCwAndCcw.HwAgOverTrvlCnt
  Set Ram Block Status1 : NxtrNvM/Set Ram Block Status  RequirementInfo="{'linktype_rmi_doors' '0000ba59 (/E-STEER Core/SubSystem Specifications/Application Functions/SF011A Learned EOT Limits)' '#SF011A_196' 'true' 'REQ:  SF011A_196' '' } %GIDa_771f18a6_b977_40f6_a8f7_f72468a6fd7f"  FuncName=Set Ram Block Status  NvMBlockName=MaxHwAgCwAndCcw  VoidFuncRtn=on  BlockChanged_DSN=NvMSRBS_BlockChanged6  Return_DSN=NvMSRBS_Return6
      settings: AttributesFormatString=%<FuncName>
  WriteFlag : Constant  RequirementInfo="{'linktype_rmi_doors' '0000ba59 (/E-STEER Core/SubSystem Specifications/Application Functions/SF011A Learned EOT Limits)' '#SF011A_196' 'true' 'REQ:  SF011A_196' '' } %GIDa_d90bada4_6107_463b_9b2c_4d1d6e8fd05d"  OutDataTypeStr=boolean
      settings: AttributesFormatString=%<OutDataTypeStr>
  wires:
  " "/1 -> Data Store Write/1
  WriteFlag/1 -> Set Ram Block Status1/1

== system SF011A_EotLrng/EotLrng/RstMaxHwAgCwAndCcw ==
  function : TriggerPort  TriggerType=function-call
  Cal1 : Constant  RequirementInfo="{'linktype_rmi_doors' '0000ba59 (/E-STEER Core/SubSystem Specifications/Application Functions/SF011A Learned EOT Limits)' '#SF011A_160' 'true' 'REQ:  SF011A_160' '' } %GIDa_3cc12535_c8b6_4d5e_b6ad_2a4eb0d50d90"  Value=0  OutDataTypeStr=single
      settings: AttributesFormatString=%<OutDataTypeStr>
  CopyRight2 : Subsystem  Description=|  mask(Copyright Information){none=on}
      | Copyright info block.                                               
      |                                                                     
      | Place copyright information at the top of every subsystem in design.
      mask prompts: none "No parameters"
      mask help: Place copyright information at the top of every subsystem in design.
      mask Display:
      | NxtrConf = 'Nexteer Confidential';
      | 
      | sys = bdroot; %handle for the current model ("system")
      | first = get_param(sys,'Created');
      | if(isempty(first))
      |     first = datestr(now,'yyyy');
      | else
      |     first = first(end-3:end);  %year is last four digits
      | end
      | 
      | last = get_param(sys,'LastModifiedDate');
      | if isempty(last)
      |     last = datestr(now,'yyyy');
      | else
      |     last = last(end-3:end);
      | end
      | 
      | if strcmp(first,last)
      |     fprintf('%s -- Copyright %s Nexteer',NxtrConf,first)
      | else
      |     fprintf('%s -- %s%s- %s Nexteer',NxtrConf,char(169),first,last)
      | end
  Reset : DataStoreWrite  RequirementInfo="{'linktype_rmi_doors' '0000ba59 (/E-STEER Core/SubSystem Specifications/Application Functions/SF011A Learned EOT Limits)' '#SF011A_160' 'true' 'REQ:  SF011A_160' '' } %GIDa_9fe432bd_bf52_4a6e_bc54_21b0d93ee9a9"  DataStoreName=MaxHwAgCwAndCcw  DataStoreElements=MaxHwAgCwAndCcw.HwAgCcwMax#MaxHwAgCwAndCcw.HwAgCwMax
  Set Ram Block Status : NxtrNvM/Set Ram Block Status  RequirementInfo="{'linktype_rmi_doors' '0000ba59 (/E-STEER Core/SubSystem Specifications/Application Functions/SF011A Learned EOT Limits)' '#SF011A_160' 'true' 'REQ:  SF011A_160' '' } %GIDa_d6a16a32_1462_4543_bef8_0d516d79e2bf"  FuncName=Set Ram Block Status  NvMBlockName=MaxHwAgCwAndCcw  VoidFuncRtn=on  BlockChanged_DSN=NvMSRBS_BlockChanged9  Return_DSN=NvMSRBS_Return9
      settings: AttributesFormatString=%<FuncName>
  WriteFlag : Constant  RequirementInfo="{'linktype_rmi_doors' '0000ba59 (/E-STEER Core/SubSystem Specifications/Application Functions/SF011A Learned EOT Limits)' '#SF011A_160' 'true' 'REQ:  SF011A_160' '' } %GIDa_bbb9b38f_b149_4e4a_85bc_da34d17daed4"  Value=true  OutDataTypeStr=boolean
      settings: AttributesFormatString=%<OutDataTypeStr>
  wires:
  Cal1/1 -> Reset/2, Reset/1
  WriteFlag/1 -> Set Ram Block Status/1

== system SF011A_EotLrng/EotLrng/RtnMaxHwAgCwAndCcw ==
  function : TriggerPort  TriggerType=function-call
  CopyRight2 : Subsystem  Description=|  mask(Copyright Information){none=on}
      | Copyright info block.                                               
      |                                                                     
      | Place copyright information at the top of every subsystem in design.
      mask prompts: none "No parameters"
      mask help: Place copyright information at the top of every subsystem in design.
      mask Display:
      | NxtrConf = 'Nexteer Confidential';
      | 
      | sys = bdroot; %handle for the current model ("system")
      | first = get_param(sys,'Created');
      | if(isempty(first))
      |     first = datestr(now,'yyyy');
      | else
      |     first = first(end-3:end);  %year is last four digits
      | end
      | 
      | last = get_param(sys,'LastModifiedDate');
      | if isempty(last)
      |     last = datestr(now,'yyyy');
      | else
      |     last = last(end-3:end);
      | end
      | 
      | if strcmp(first,last)
      |     fprintf('%s -- Copyright %s Nexteer',NxtrConf,first)
      | else
      |     fprintf('%s -- %s%s- %s Nexteer',NxtrConf,char(169),first,last)
      | end
  Data Store Read6 : DataStoreRead  RequirementInfo="{'linktype_rmi_doors' '0000ba59 (/E-STEER Core/SubSystem Specifications/Application Functions/SF011A Learned EOT Limits)' '#SF011A_161' 'true' 'REQ:  SF011A_161' '' } %GIDa_79990203_d58d_4a4c_bb9e_48ed75722783"  DataStoreName=MaxHwAgCwAndCcw  DataStoreElements=MaxHwAgCwAndCcw.HwAgCcwMax#MaxHwAgCwAndCcw.HwAgCwMax
  HwAgCcwMax : Outport  RequirementInfo="{'linktype_rmi_doors' '0000ba59 (/E-STEER Core/SubSystem Specifications/Application Functions/SF011A Learned EOT Limits)' '#SF011A_161' 'true' 'REQ:  SF011A_161' '' } %GIDa_ec7f4f7e_251a_40ec_af61_4b6c06d4a4bf"
  HwAgCwMax : Outport  RequirementInfo="{'linktype_rmi_doors' '0000ba59 (/E-STEER Core/SubSystem Specifications/Application Functions/SF011A Learned EOT Limits)' '#SF011A_161' 'true' 'REQ:  SF011A_161' '' } %GIDa_69e86fcc_cbdc_4266_a80c_53eb8063d5c7"  Port=2
  wires:
  Data Store Read6/1 -> HwAgCcwMax/1
  Data Store Read6/2 -> HwAgCwMax/1

== system SF011A_EotLrng/EotLrng/SerlComRstEot ==
  function : TriggerPort  TriggerType=function-call
  Calibration4 : Constant  RequirementInfo="{'linktype_rmi_doors' '0000ba59 (/E-STEER Core/SubSystem Specifications/Application Functions/SF011A Learned EOT Limits)' '#SF011A_122' 'true' 'REQ:  SF011A_122' '' } %GIDa_fbd95297_23b1_43fe_97fc_157122b2bd6a"  Value=EotProtnRackTrvlLimrEna
  CopyRight2 : Subsystem  Description=|  mask(Copyright Information){none=on}
      | Copyright info block.                                               
      |                                                                     
      | Place copyright information at the top of every subsystem in design.
      mask prompts: none "No parameters"
      mask help: Place copyright information at the top of every subsystem in design.
      mask Display:
      | NxtrConf = 'Nexteer Confidential';
      | 
      | sys = bdroot; %handle for the current model ("system")
      | first = get_param(sys,'Created');
      | if(isempty(first))
      |     first = datestr(now,'yyyy');
      | else
      |     first = first(end-3:end);  %year is last four digits
      | end
      | 
      | last = get_param(sys,'LastModifiedDate');
      | if isempty(last)
      |     last = datestr(now,'yyyy');
      | else
      |     last = last(end-3:end);
      | end
      | 
      | if strcmp(first,last)
      |     fprintf('%s -- Copyright %s Nexteer',NxtrConf,first)
      | else
      |     fprintf('%s -- %s%s- %s Nexteer',NxtrConf,char(169),first,last)
      | end
  If : If  RequirementInfo="{'linktype_rmi_doors' '0000ba59 (/E-STEER Core/SubSystem Specifications/Application Functions/SF011A Learned EOT Limits)' '#SF011A_122' 'true' 'REQ:  SF011A_122' '' } %GIDa_fa50ba8b_fd76_4c98_9bf4_f9c82f98754d"  IfExpression=~u1  ShowElse=off
  SetRstLimReq : Subsystem  RequirementInfo="{'linktype_rmi_doors' '0000ba59 (/E-STEER Core/SubSystem Specifications/Application Functions/SF011A Learned EOT Limits)' '#SF011A_122' 'true' 'REQ:  SF011A_122' '' } %GIDa_a7c0bb26_2cc6_4d83_a4be_255c23d3cef9"  TreatAsAtomicUnit=on
  wires:
  Calibration4/1 -> If/1
  If/1 -> SetRstLimReq/Action

== system SF011A_EotLrng/EotLrng/SetHwAgOverTrvlCnt ==
  HwAgOverTrvlCnt : Inport  RequirementInfo="{'linktype_rmi_doors' '0000ba59 (/E-STEER Core/SubSystem Specifications/Application Functions/SF011A Learned EOT Limits)' '#SF011A_201' 'true' 'REQ:  SF011A_201' '' } %GIDa_517bd9c2_4b83_4dc3_a5d4_2473b3d80d59"
  function : TriggerPort  TriggerType=function-call
  CopyRight2 : Subsystem  Description=|  mask(Copyright Information){none=on}
      | Copyright info block.                                               
      |                                                                     
      | Place copyright information at the top of every subsystem in design.
      mask prompts: none "No parameters"
      mask help: Place copyright information at the top of every subsystem in design.
      mask Display:
      | NxtrConf = 'Nexteer Confidential';
      | 
      | sys = bdroot; %handle for the current model ("system")
      | first = get_param(sys,'Created');
      | if(isempty(first))
      |     first = datestr(now,'yyyy');
      | else
      |     first = first(end-3:end);  %year is last four digits
      | end
      | 
      | last = get_param(sys,'LastModifiedDate');
      | if isempty(last)
      |     last = datestr(now,'yyyy');
      | else
      |     last = last(end-3:end);
      | end
      | 
      | if strcmp(first,last)
      |     fprintf('%s -- Copyright %s Nexteer',NxtrConf,first)
      | else
      |     fprintf('%s -- %s%s- %s Nexteer',NxtrConf,char(169),first,last)
      | end
  Data Store Write : DataStoreWrite  RequirementInfo="{'linktype_rmi_doors' '0000ba59 (/E-STEER Core/SubSystem Specifications/Application Functions/SF011A Learned EOT Limits)' '#SF011A_201' 'true' 'REQ:  SF011A_201' '' } %GIDa_0d03781f_d2c5_4ce4_a041_dbc09c32d4e5"  DataStoreName=MaxHwAgCwAndCcw  DataStoreElements=MaxHwAgCwAndCcw.HwAgOverTrvlCnt
  Set Ram Block Status1 : NxtrNvM/Set Ram Block Status  RequirementInfo="{'linktype_rmi_doors' '0000ba59 (/E-STEER Core/SubSystem Specifications/Application Functions/SF011A Learned EOT Limits)' '#SF011A_201' 'true' 'REQ:  SF011A_201' '' } %GIDa_275738a2_1780_411a_a83f_8c932bf7f65e"  FuncName=Set Ram Block Status  NvMBlockName=MaxHwAgCwAndCcw  VoidFuncRtn=on  BlockChanged_DSN=NvMSRBS_BlockChanged5  Return_DSN=NvMSRBS_Return5
      settings: AttributesFormatString=%<FuncName>
  WriteFlag : Constant  RequirementInfo="{'linktype_rmi_doors' '0000ba59 (/E-STEER Core/SubSystem Specifications/Application Functions/SF011A Learned EOT Limits)' '#SF011A_201' 'true' 'REQ:  SF011A_201' '' } %GIDa_1916b4fc_55f8_49dc_9459_a256adc9c68d"  OutDataTypeStr=boolean
      settings: AttributesFormatString=%<OutDataTypeStr>
  wires:
  HwAgOverTrvlCnt/1 -> Data Store Write/1
  WriteFlag/1 -> Set Ram Block Status1/1

== system SF011A_EotLrng/call_EotLrngInit1/CopyRight2 ==

== system SF011A_EotLrng/call_EotLrngPer1/CopyRight2 ==

== system SF011A_EotLrng/EotLrng/EotLrngInit1/CopyRight2 ==

== system SF011A_EotLrng/EotLrng/EotLrngInit1/NvmNotOk ==
  Action Port : ActionPort  ActionType=then
  Cal1 : Constant  RequirementInfo="{'linktype_rmi_doors' '0000ba59 (/E-STEER Core/SubSystem Specifications/Application Functions/SF011A Learned EOT Limits)' '#SF011A_124' 'true' 'REQ:  SF011A_124' '' } %GIDa_78f2c12b_62b3_4003_88e8_c07dd8af146c"  Value=0  OutDataTypeStr=single
  CopyRight2 : Subsystem  Description=|  mask(Copyright Information){none=on}
      | Copyright info block.                                               
      |                                                                     
      | Place copyright information at the top of every subsystem in design.
      mask prompts: none "No parameters"
      mask help: Place copyright information at the top of every subsystem in design.
      mask Display:
      | NxtrConf = 'Nexteer Confidential';
      | 
      | sys = bdroot; %handle for the current model ("system")
      | first = get_param(sys,'Created');
      | if(isempty(first))
      |     first = datestr(now,'yyyy');
      | else
      |     first = first(end-3:end);  %year is last four digits
      | end
      | 
      | last = get_param(sys,'LastModifiedDate');
      | if isempty(last)
      |     last = datestr(now,'yyyy');
      | else
      |     last = last(end-3:end);
      | end
      | 
      | if strcmp(first,last)
      |     fprintf('%s -- Copyright %s Nexteer',NxtrConf,first)
      | else
      |     fprintf('%s -- %s%s- %s Nexteer',NxtrConf,char(169),first,last)
      | end
  Reset : DataStoreWrite  RequirementInfo="{'linktype_rmi_doors' '0000ba59 (/E-STEER Core/SubSystem Specifications/Application Functions/SF011A Learned EOT Limits)' '#SF011A_124' 'true' 'REQ:  SF011A_124' '' } %GIDa_15b67e1e_5f43_4b38_96f1_f27ff78bfcf3"  DataStoreName=MaxHwAgCwAndCcw  DataStoreElements=MaxHwAgCwAndCcw.HwAgCcwMax#MaxHwAgCwAndCcw.HwAgCwMax
  Set Ram Block Status : NxtrNvM/Set Ram Block Status  RequirementInfo="{'linktype_rmi_doors' '0000ba59 (/E-STEER Core/SubSystem Specifications/Application Functions/SF011A Learned EOT Limits)' '#SF011A_124' 'true' 'REQ:  SF011A_124' '' } %GIDa_fdf2728b_1b84_471a_9422_29bbe63787e7"  FuncName=Set Ram Block Status  NvMBlockName=MaxHwAgCwAndCcw  VoidFuncRtn=on  BlockChanged_DSN=NvMSRBS_BlockChanged4  Return_DSN=NvMSRBS_Return4
      settings: AttributesFormatString=%<FuncName>
  WriteFlag : Constant  RequirementInfo="{'linktype_rmi_doors' '0000ba59 (/E-STEER Core/SubSystem Specifications/Application Functions/SF011A Learned EOT Limits)' '#SF011A_124' 'true' 'REQ:  SF011A_124' '' } %GIDa_4c9ca891_7671_4ff7_b93f_3561c3afee1c"  Value=true  OutDataTypeStr=boolean
      settings: AttributesFormatString=%<OutDataTypeStr>
  wires:
  Cal1/1 -> Reset/2, Reset/1
  WriteFlag/1 -> Set Ram Block Status/1
